simulink model "Helikopter"  (R2017b)
settings: Solver=ode5  StartTime=0.0  StopTime=Inf  FixedStep=0.001  RelTol=1e-3  AbsTol=1e-6
values from neighbouring files (symbols this model uses):
  wsp_V = polyfit(vp, napiecie, 1)    [Helicopter_main.m]    (also in Helicopter_main_test.m)
undefined symbols (not defined in the file or in its folder): RTDAC4PCIBaseAddress
libraries: simulink x3
settings Model: SimulationMode=external  ExtModeTrigDuration=120000  ExtModeTrigLevel=0.400000  Creator=jims  LastModifiedBy=Marcin
settings DataIOCC: ExternalInput=[]  InitialState=[]  MaxDataPoints=5000  SaveFormat=Array  SignalLoggingSaveFormat=ModelDataLogs  SaveOutput=off  SaveTime=off  SignalLoggingName=sigsOut
settings OptimizationCC: BooleanDataType=off  ExpressionDepthLimit=2147483647  InitFltsAndDblsToZero=on
settings DebuggingCC: SaveWithParameterizedLinksMsg=none  UnderspecifiedInitializationDetection=Classic  MergeDetectMultiDrivingBlocksExec=none  SignalResolutionControl=TryResolveAllWithWarning  MultiTaskDSMMsg=warning  MultiTaskCondExecSysMsg=none  IntegerOverflowMsg=none  FcnCallInpInsideContextMsg=warning  StateNameClashWarn=warning  SFUnexpectedBacktrackingDiag=warning  SFNoUnconditionalDefaultTransitionDiag=warning  SFExecutionAtInitializationDiag=none  IntegerSaturationMsg=none
settings HardwareCC: TargetBitPerLong=64  TargetBitPerPointer=64  TargetIntDivRoundTo=Zero  TargetEndianess=LittleEndian  TargetWordSize=64  TargetHWDeviceType=Intel->x86-64
settings ModelReferenceCC: PropagateSignalLabelsOutOfModel=off
settings RTWCC: SystemTargetFile=sldrt.tlc  TemplateMakefile=sldrt.tmf  Description=Simulink Desktop Real-Time  RTWCompilerOptimization=on
settings CodeAppCC: MaxIdLength=95  StateflowObjectComments=on
settings SimulinkDesktopRealTimeCC: TargetPreCompLibLocation=C:\MATLAB\R2017b\toolbox\sldrt\lib\win64  TargetLangStandard=C89/C90 (ANSI)  ModelReferenceCompliant=off  CompOptLevelCompliant=off  SupportVariableSizeSignals=off
settings ConfigComp: CovMetricSettings=dw  CovHtmlReporting=on  CovSaveCumulativeToWorkspaceVar=on  CovSaveSingleToWorkspaceVar=on  CovExternalEMLEnable=off

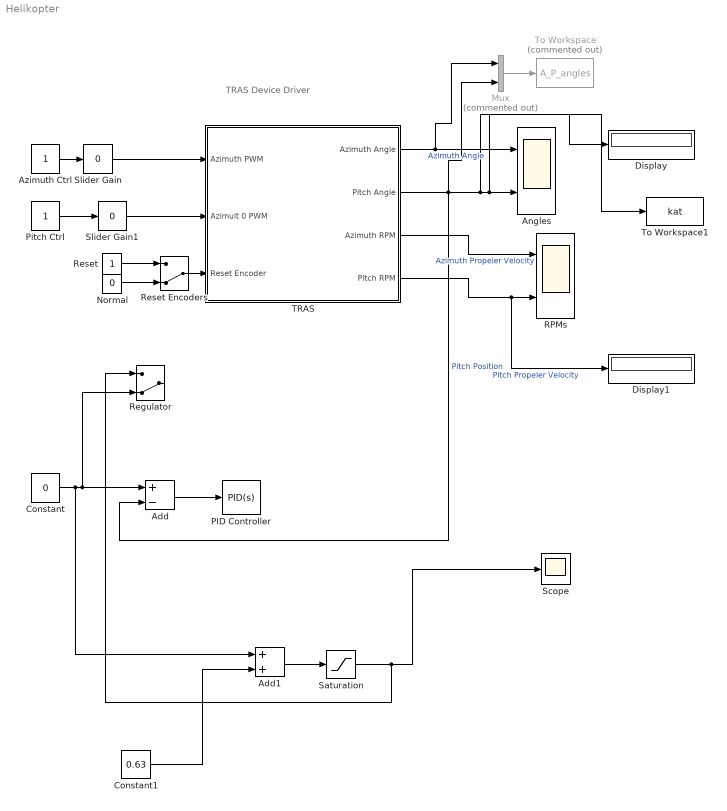
== system Helikopter ==
  note: TRAS Device Driver
  Add : Sum  Inputs=+-
  Add1 : Sum
  Angles : Scope  NumInputPorts=2
  Azimuth Ctrl : Constant  SampleTime=-1
  Constant : Constant  Value=0
  Constant1 : Constant  Value=0.63
  Display : Display
  Display1 : Display
  Mux : Mux  Commented=on  Inputs=2
  Normal : Constant  Value=0
  PID Controller : simulink/Continuous/PID Controller  Controller=PID  TimeDomain=Continuous-time  SampleTime=-1  IntegratorMethod=Forward Euler  FilterMethod=Forward Euler  Form=Parallel  UseFilter=on  ControllerParametersSource=internal  P=0.01  I=0  D=0  N=100  InitialConditionSource=internal  InitialConditionForIntegrator=0  InitialConditionForFilter=0  ExternalReset=none  LimitOutput=on  UpperSaturationLimit=1  LowerSaturationLimit=-1  LinearizeAsGain=on  AntiWindupMode=none  Kb=1  TrackingMode=off  Kt=1  PParamMin=[]  PParamMax=[]  IParamMin=[]  IParamMax=[]  DParamMin=[]  DParamMax=[]  NParamMin=[]  NParamMax=[]  KbParamMin=[]  KbParamMax=[]  KtParamMin=[]  KtParamMax=[]  POutMin=[]  POutMax=[]  IOutMin=[]  IOutMax=[]  DOutMin=[]  DOutMax=[]  NOutMin=[]  NOutMax=[]  KbOutMin=[]  KbOutMax=[]  KtOutMin=[]  KtOutMax=[]  IntegratorOutMin=[]  IntegratorOutMax=[]  FilterOutMin=[]  FilterOutMax=[]  SumOutMin=[]  SumOutMax=[]  SumI1OutMin=[]  SumI1OutMax=[]  SumI2OutMin=[]  SumI2OutMax=[]  SumI3OutMin=[]  SumI3OutMax=[]  SumDOutMin=[]  SumDOutMax=[]  SaturationOutMin=[]  SaturationOutMax=[]  IntegratorContinuousStateAttributes=''  IntegratorStateMustResolveToSignalObject=off  IntegratorRTWStateStorageClass=Auto  FilterContinuousStateAttributes=''  FilterStateMustResolveToSignalObject=off  FilterRTWStateStorageClass=Auto  DifferentiatorICPrevScaledInput=0  DifferentiatorOutMin=[]  DifferentiatorOutMax=[]  InitialConditionSetting=State (most efficient)  FilterDiffOutCoefMin=[]  FilterDiffOutCoefMax=[]  SumDenOutMin=[]  SumDenOutMax=[]  SumNumOutMin=[]  SumNumOutMax=[]  ReciprocalOutMin=[]  ReciprocalOutMax=[]  DivideOutMin=[]  DivideOutMax=[]  TunerSelectOption=Transfer Function Based (PID Tuner App)
  Pitch Ctrl : Constant  SampleTime=-1
  RPMs : Scope  NumInputPorts=2
  Regulator : ManualSwitch  CurrentSetting=0
  Reset : Constant
  Reset Encoders : ManualSwitch  CurrentSetting=0
  Saturation : Saturate  UpperLimit=1  LowerLimit=-1
  Scope : Scope
  Slider Gain : simulink/Math Operations/Slider Gain  gain=0  low=-1  high=1
  Slider Gain1 : simulink/Math Operations/Slider Gain  gain=0  low=-1  high=1
  TRAS : Subsystem  mask{BaseAddress=RTDAC4PCIBaseAddress, T0=0.001}
      mask prompts: BaseAddress "Base Address:"; T0 "Sampling Period:"
      mask Display: image(imread('TRAS.JPG'))
  To Workspace : ToWorkspace  Commented=on  VariableName=A_P_angles  SampleTime=-1
  To Workspace1 : ToWorkspace  VariableName=kat  SampleTime=-1
  wires:
  TRAS/1(Azimuth Angle) -> Mux/1, Angles/1  "Azimuth Angle"
  TRAS/2(Pitch Angle) -> Add/2, Mux/2, To Workspace1/1, Display/1, Angles/2  "Pitch Position"
  Azimuth Ctrl/1 -> Slider Gain/1
  TRAS/3(Azimuth RPM) -> RPMs/1  "Azimuth Propeler Velocity"
  TRAS/4(Pitch RPM) -> Display1/1, RPMs/2  "Pitch Propeler Velocity"
  Normal/1 -> Reset Encoders/2
  Reset/1 -> Reset Encoders/1
  Reset Encoders/1 -> TRAS/3(Reset Encoder)
  Pitch Ctrl/1 -> Slider Gain1/1
  Slider Gain/1 -> TRAS/1(Azimuth PWM)
  Mux/1 -> To Workspace/1
  Constant/1 -> Add1/1, Regulator/2, Add/1
  Add/1 -> PID Controller/1
  Add1/1 -> Saturation/1
  Constant1/1 -> Add1/2
  Saturation/1 -> Regulator/1, Scope/1
  Slider Gain1/1 -> TRAS/2(Azimult 0 PWM)

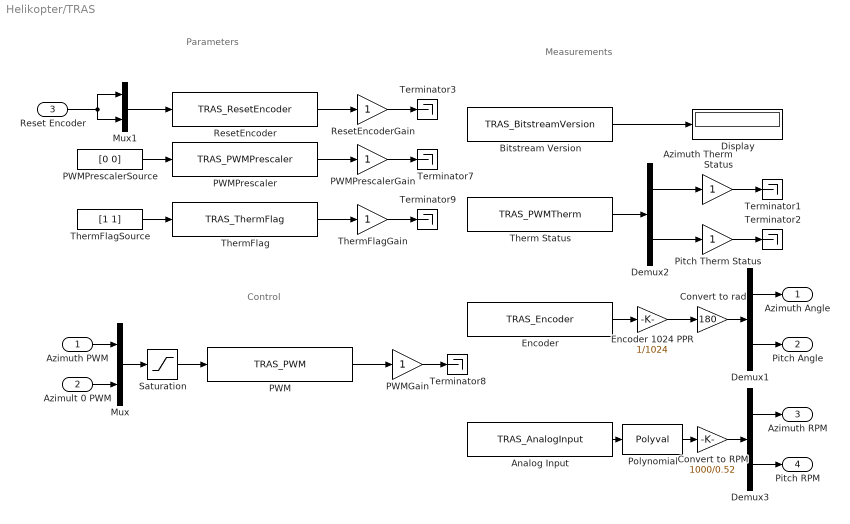
== system Helikopter/TRAS ==
  note: Parameters
  note: Control
  note: Measurements
  Azimuth PWM : Inport
  Azimult 0 PWM : Inport  Port=2
  Reset Encoder : Inport  Port=3
  Analog Input : S-Function  FunctionName=TRAS_AnalogInput  Parameters=BaseAddress, [1 0], [1 1], T0  SFunctionDeploymentMode=off  EnableBusSupport=off
  Azimuth Therm Status : Gain  SaturateOnIntegerOverflow=on  OutDataTypeStr=Inherit: Same as input  ParamDataTypeStr=Inherit: Same as input
  Bitstream Version : S-Function  FunctionName=TRAS_BitstreamVersion  Parameters=BaseAddress, T0  SFunctionDeploymentMode=off  EnableBusSupport=off
  Convert to RPM : Gain  Gain=1000/0.52  SaturateOnIntegerOverflow=on  OutDataTypeStr=Inherit: Same as input  ParamDataTypeStr=Inherit: Same as input
  Convert to rad : Gain  Gain=180  SaturateOnIntegerOverflow=on  OutDataTypeStr=Inherit: Same as input  ParamDataTypeStr=Inherit: Same as input
  Demux1 : Demux  Outputs=2
  Demux2 : Demux  Outputs=2
  Demux3 : Demux  Outputs=2
  Display : Display
  Encoder : S-Function  FunctionName=TRAS_Encoder  Parameters=BaseAddress, T0  SFunctionDeploymentMode=off  EnableBusSupport=off
  Encoder 1024 PPR : Gain  Gain=1/1024  SaturateOnIntegerOverflow=on  OutDataTypeStr=Inherit: Same as input  ParamDataTypeStr=Inherit: Same as input
  Mux : Mux  Inputs=2
  Mux1 : Mux  Inputs=2
  PWM : S-Function  FunctionName=TRAS_PWM  Parameters=BaseAddress, T0  SFunctionDeploymentMode=off  EnableBusSupport=off
  PWMGain : Gain  SaturateOnIntegerOverflow=on  OutDataTypeStr=Inherit: Same as input  ParamDataTypeStr=Inherit: Same as input
  PWMPrescaler : S-Function  FunctionName=TRAS_PWMPrescaler  Parameters=BaseAddress, T0  SFunctionDeploymentMode=off  EnableBusSupport=off
  PWMPrescalerGain : Gain  SaturateOnIntegerOverflow=on  OutDataTypeStr=Inherit: Same as input  ParamDataTypeStr=Inherit: Same as input
  PWMPrescalerSource : Constant  Value=[0 0]
  Pitch Therm Status : Gain  SaturateOnIntegerOverflow=on  OutDataTypeStr=Inherit: Same as input  ParamDataTypeStr=Inherit: Same as input
  Polynomial : Polyval  Coefs=wsp_V
  ResetEncoder : S-Function  FunctionName=TRAS_ResetEncoder  Parameters=BaseAddress, T0  SFunctionDeploymentMode=off  EnableBusSupport=off
  ResetEncoderGain : Gain  SaturateOnIntegerOverflow=on  OutDataTypeStr=Inherit: Same as input  ParamDataTypeStr=Inherit: Same as input
  Saturation : Saturate  UpperLimit=1  LowerLimit=-1
  Terminator{1..3,7..9} (6 alike) : Terminator
  Therm Status : S-Function  FunctionName=TRAS_PWMTherm  Parameters=BaseAddress, T0  SFunctionDeploymentMode=off  EnableBusSupport=off
  "ThermFlag " : S-Function  FunctionName=TRAS_ThermFlag  Parameters=BaseAddress, T0  SFunctionDeploymentMode=off  EnableBusSupport=off
  ThermFlagGain : Gain  SaturateOnIntegerOverflow=on  OutDataTypeStr=Inherit: Same as input  ParamDataTypeStr=Inherit: Same as input
  ThermFlagSource : Constant  Value=[1 1]
  Azimuth Angle : Outport  InitialOutput=0
  Pitch Angle : Outport  Port=2  InitialOutput=0
  Azimuth RPM : Outport  Port=3  InitialOutput=0
  Pitch RPM : Outport  Port=4  InitialOutput=0
  wires:
  Encoder 1024 PPR/1 -> Convert to rad/1
  Encoder/1 -> Encoder 1024 PPR/1
  Saturation/1 -> PWM/1
  Mux/1 -> Saturation/1
  PWM/1 -> PWMGain/1
  PWMGain/1 -> Terminator8/1
  ResetEncoder/1 -> ResetEncoderGain/1
  PWMPrescaler/1 -> PWMPrescalerGain/1
  Mux1/1 -> ResetEncoder/1
  PWMPrescalerSource/1 -> PWMPrescaler/1
  ResetEncoderGain/1 -> Terminator3/1
  PWMPrescalerGain/1 -> Terminator7/1
  Azimult 0 PWM/1 -> Mux/2
  Azimuth PWM/1 -> Mux/1
  Demux1/2 -> Pitch Angle/1
  Convert to rad/1 -> Demux1/1
  Demux1/1 -> Azimuth Angle/1
  Therm Status/1 -> Demux2/1
  Demux2/2 -> Pitch Therm Status/1
  Demux2/1 -> Azimuth Therm Status/1
  Azimuth Therm Status/1 -> Terminator1/1
  Pitch Therm Status/1 -> Terminator2/1
  Bitstream Version/1 -> Display/1
  Analog Input/1 -> Polynomial/1
  Demux3/2 -> Pitch RPM/1
  Demux3/1 -> Azimuth RPM/1
  Reset Encoder/1 -> Mux1/1, Mux1/2
  "ThermFlag "/1 -> ThermFlagGain/1
  ThermFlagSource/1 -> "ThermFlag "/1
  ThermFlagGain/1 -> Terminator9/1
  Polynomial/1 -> Convert to RPM/1
  Convert to RPM/1 -> Demux3/1
